simulink model "fixed_graph_sim_lpv"  (R2022b)
settings: Solver=VariableStepAuto  StartTime=0.0  StopTime=80  RelTol=1e-3
values from neighbouring files (symbols this model uses):
  A = [0 1 0; 0 0 1; 0 0 -1/tau]    [cacc_consensus_main.m]    (also in dyn_graph.m; dyn_graph_10.m; dyn_graph_10_disturb.m; fixed_graph.m)
  B = [0 0 1/tau]'    [cacc_consensus_main.m]    (also in dyn_graph.m; dyn_graph_10.m; dyn_graph_10_disturb.m; fixed_graph.m)
  C = diag([1 1 1])    [cacc_consensus_main.m]    (also in dyn_graph.m; dyn_graph_10.m; dyn_graph_10_disturb.m; fixed_graph.m)
  D = [0 0 0]'    [cacc_consensus_main.m]    (also in dyn_graph.m; dyn_graph_10.m; dyn_graph_10_disturb.m; fixed_graph.m)
  h = 1    [cacc_consensus_main.m]    (also in dyn_graph.m; dyn_graph_10.m; dyn_graph_10_disturb.m; fixed_graph.m)
  K_cacc = K_lqr    [cacc_consensus_main.m]    (also in dyn_graph.m = -K_lmi; fixed_graph.m = -K_lmi; fixed_graph_lpv.m = -K_lmi)
  lv = 4.46    [cacc_consensus_main.m]    (also in dyn_graph.m; dyn_graph_10.m; dyn_graph_10_disturb.m; fixed_graph.m)
  q0_init = 0    [cacc_consensus_main.m]    (also in dyn_graph.m; dyn_graph_10.m = rand() * range; dyn_graph_10_disturb.m = rand() * range; fixed_graph.m = rand() * range)
  q1_init = 0    [cacc_consensus_main.m]    (also in dyn_graph.m; dyn_graph_10.m = rand() * range; dyn_graph_10_disturb.m = rand() * range; fixed_graph.m = rand() * range)
  q2_init = 0    [cacc_consensus_main.m]    (also in dyn_graph.m; dyn_graph_10.m = rand() * range; dyn_graph_10_disturb.m = rand() * range; fixed_graph.m = rand() * range)
  q3_init = 0    [cacc_consensus_main.m]    (also in dyn_graph.m; dyn_graph_10.m = rand() * range; dyn_graph_10_disturb.m = rand() * range; fixed_graph.m = rand() * range)
  rv = 0    [cacc_consensus_main.m]    (also in dyn_graph.m; dyn_graph_10.m; dyn_graph_10_disturb.m; fixed_graph.m)
  tau = 0.1    [cacc_consensus_main.m]    (also in dyn_graph.m; dyn_graph_10.m; dyn_graph_10_disturb.m; fixed_graph.m)
libraries: cstblocks x4, simulink x2
settings Model: Creator=phatdo  LastModifiedBy=phatdo
settings DataIOCC: ReturnWorkspaceOutputs=off

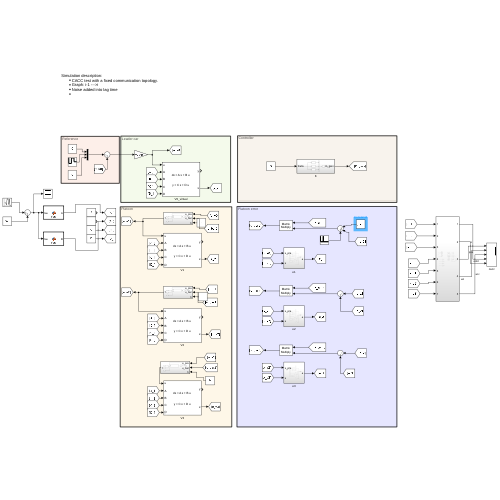
[thumbnail: Simulink's stored preview of the top-level diagram]
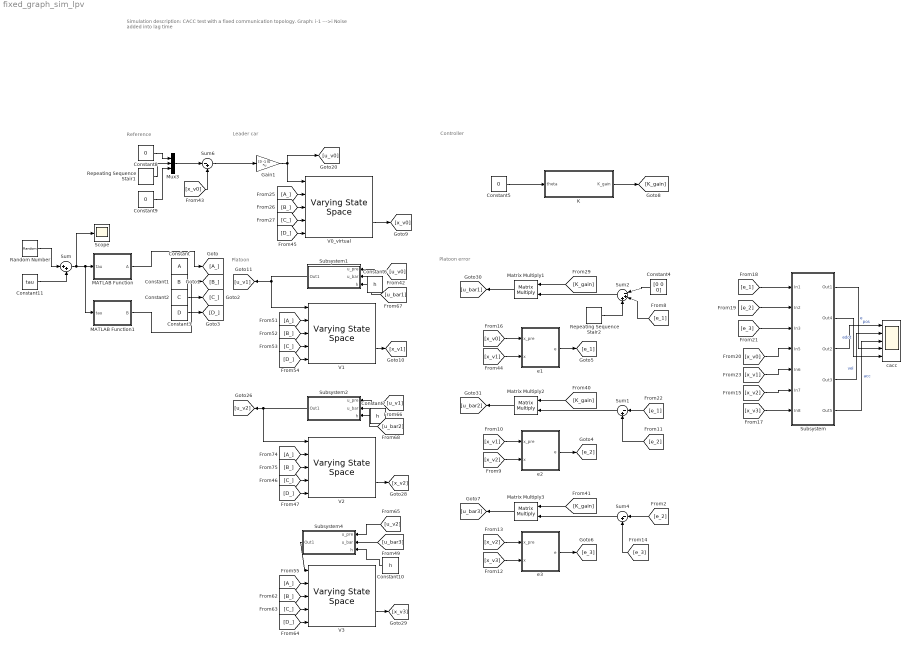
== system fixed_graph_sim_lpv ==
  note: Reference
  note: Controller
  note: Leader car
  note: Platoon
  note: Platoon error
  note: Simulation description:
      | CACC test with a fixed communication topology.
      | Graph: i-1 --->i
      | Noise added into lag time
  Constant : Constant  Value=A
  Constant1 : Constant  Value=B
  Constant10 : Constant  Value=h
  Constant11 : Constant  Value=tau
  Constant2 : Constant  Value=C
  Constant3 : Constant  Value=D
  Constant4 : Constant  Value=[0 0 0]
  Constant5 : Constant  Value=0
  Constant6 : Constant  Value=h
  Constant7 : Constant  Value=h
  Constant8 : Constant  Value=0
  Constant9 : Constant  Value=0
  Gain1 : Gain  Gain=[0 -1 0]  Multiplication=Matrix(K*u) (u vector)
  K : Subsystem
  MATLAB Function : MATLAB Function  TreatAsAtomicUnit=on
  MATLAB Function1 : MATLAB Function  TreatAsAtomicUnit=on
  Matrix Multiply1 : Product  Multiplication=Matrix(*)
  Matrix Multiply2 : Product  Multiplication=Matrix(*)
  Matrix Multiply3 : Product  Multiplication=Matrix(*)
  Mux3 : Mux  Inputs=3
  Random Number : RandomNumber  Variance=0.0001  SampleTime=1
  Repeating Sequence Stair1 : simulink/Sources/Repeating Sequence Stair  OutValues=[5 20 10]  tsamp=20  OutMin=[]  OutMax=[]  OutDataTypeStr=double  OutputDataTypeScalingMode=double  OutDataType=fixdt(0,8)  ConRadixGroup=Best Precision: Vector-wise  OutScaling=2^-12
  Repeating Sequence Stair2 : simulink/Sources/Repeating Sequence Stair  OutValues=[0 0 0 0 0 0 1 0 0 0 0 0 0 0 0 0 0 0].'  tsamp=5  OutMin=[]  OutMax=[]  OutDataTypeStr=double  OutputDataTypeScalingMode=double  OutDataType=fixdt(0,8)  ConRadixGroup=Best Precision: Vector-wise  OutScaling=2^-12
  Scope : Scope
  Subsystem : Subsystem
  Subsystem1 : Subsystem
  Subsystem2 : Subsystem
  Subsystem4 : Subsystem
  Sum : Sum  Inputs=|++
  Sum1 : Sum  Inputs=|-+
  Sum2 : Sum  Inputs=|-++
  Sum4 : Sum  Inputs=|-+
  Sum6 : Sum  Inputs=|-+
  V0_virtual : cstblocks/Linear Parameter Varying/Varying State Space  x0=[q0_init;0;0]  xNames=''  OutputX=on  OutputDX=off
  V1 : cstblocks/Linear Parameter Varying/Varying State Space  x0=[q1_init;0;0]  xNames=''  OutputX=on  OutputDX=off
  V2 : cstblocks/Linear Parameter Varying/Varying State Space  x0=[q2_init;0;0]  xNames=''  OutputX=on  OutputDX=off
  V3 : cstblocks/Linear Parameter Varying/Varying State Space  x0=[q3_init ;0 ; 0]  xNames=''  OutputX=on  OutputDX=off
  cacc : Scope  NumInputPorts=5
  e1 : Subsystem
  e2 : Subsystem
  e3 : Subsystem
  wires:
  Sum2/1 -> Matrix Multiply1/2
  Sum1/1 -> Matrix Multiply2/2
  Constant2/1 -> [C_]
  Constant3/1 -> [D_]
  Constant5/1 -> K/1(theta)
  K/1(K_gain) -> [K_gain]
  [K_gain] -> Matrix Multiply1/1
  [K_gain] -> Matrix Multiply2/1
  [K_gain] -> Matrix Multiply3/1
  Sum4/1 -> Matrix Multiply3/2
  Repeating Sequence Stair1/1 -> Mux3/2
  [A_] -> V1/2
  [C_] -> V1/4
  [D_] -> V0_virtual/5
  V0_virtual/2 -> [x_v0]
  [B_] -> V0_virtual/3
  [A_] -> V0_virtual/2
  V1/2 -> [x_v1]
  Constant9/1 -> Mux3/3
  Constant8/1 -> Mux3/1
  [x_v0] -> Sum6/2
  [C_] -> V0_virtual/4
  [B_] -> V1/3
  Sum6/1 -> Gain1/1
  [D_] -> V3/5
  V3/2 -> [x_v3]
  [A_] -> V3/2
  [B_] -> V3/3
  [u_v1] -> Subsystem2/1(u_pre)
  [C_] -> V2/4
  V2/2 -> [x_v2]
  [D_] -> V2/5
  [C_] -> V3/4
  [A_] -> V2/2
  [B_] -> V2/3
  [x_v0] -> Subsystem/4(In5)
  [x_v1] -> Subsystem/5(In6)
  [x_v2] -> Subsystem/6(In7)
  [x_v3] -> Subsystem/7(In8)
  Subsystem/1(Out1) -> cacc/4  "e"
  Subsystem/3(Out2) -> cacc/1  "pos"
  Subsystem/4(Out3) -> cacc/2  "vel"
  Gain1/1 -> V0_virtual/1, [u_v0]
  Mux3/1 -> Sum6/1
  [u_v0] -> Subsystem1/1(u_pre)
  [u_bar1] -> Subsystem1/2(u_bar)
  [x_v0] -> e1/1(x_pre)
  [x_v1] -> e1/2(x)
  e1/1(e) -> [e_1]
  [e_1] -> Sum2/2
  [x_v1] -> e2/1(x_pre)
  e2/1(e) -> [e_2]
  [x_v2] -> e2/2(x)
  [e_2] -> Sum1/2
  e3/1(e) -> [e_3]
  [x_v3] -> e3/2(x)
  [e_3] -> Sum4/2
  [e_1] -> Subsystem/1(In1)
  [e_2] -> Subsystem/2(In2)
  [e_3] -> Subsystem/3(In3)
  [e_1] -> Sum1/1
  Constant4/1 -> Sum2/1
  Subsystem/2(Out4) -> cacc/5  "edot"
  [D_] -> V1/5
  Subsystem/5(Out5) -> cacc/3  "acc"
  Sum/1 -> Scope/1, MATLAB Function1/1(tau), MATLAB Function/1(tau)
  [u_bar3] -> Subsystem4/2(u_bar)
  [u_v2] -> Subsystem4/1(u_pre)
  [u_bar2] -> Subsystem2/2(u_bar)
  Constant6/1 -> Subsystem1/3(h)
  Constant7/1 -> Subsystem2/3(h)
  Constant10/1 -> Subsystem4/3(h)
  [x_v2] -> e3/1(x_pre)
  Constant11/1 -> Sum/2
  Random Number/1 -> Sum/1
  [e_2] -> Sum4/1
  Matrix Multiply1/1 -> [u_bar1]
  Matrix Multiply2/1 -> [u_bar2]
  Matrix Multiply3/1 -> [u_bar3]
  Subsystem1/1(Out1) -> V1/1, [u_v1]
  Subsystem2/1(Out1) -> V2/1, [u_v2]
  Subsystem4/1(Out1) -> V3/1
  MATLAB Function/1(A) -> [A_]
  MATLAB Function1/1(B) -> [B_]
  Repeating Sequence Stair2/1 -> Sum2/3

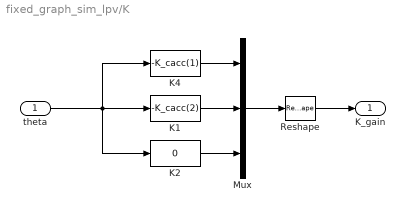
== system fixed_graph_sim_lpv/K ==
  theta : Inport
  K1 : Fcn  Expr=-K_cacc(2)
  K2 : Fcn  Expr=0
  K4 : Fcn  Expr=-K_cacc(1)
  Mux : Mux  Inputs=3
  Reshape : Reshape  OutputDimensionality=Customize  OutputDimensions=[1,3]
  K_gain : Outport
  wires:
  Mux/1 -> Reshape/1
  Reshape/1 -> K_gain/1
  K4/1 -> Mux/1
  K1/1 -> Mux/2
  K2/1 -> Mux/3
  theta/1 -> K2/1, K1/1, K4/1

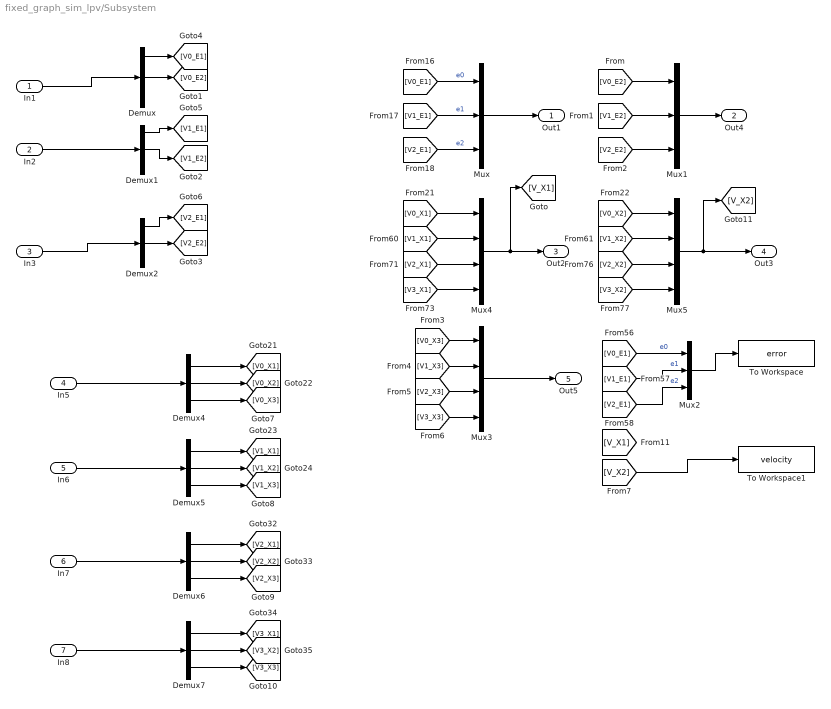
== system fixed_graph_sim_lpv/Subsystem ==
  In1 : Inport
  In2 : Inport  Port=2
  In3 : Inport  Port=3
  In5 : Inport  Port=4
  In6 : Inport  Port=5
  In7 : Inport  Port=6
  In8 : Inport  Port=7
  Demux{,1..2,4..7} (7 alike) : Demux  Outputs=3
  Mux : Mux  Inputs=3
  Mux1 : Mux  Inputs=3
  Mux2 : Mux  Inputs=3
  Mux3 : Mux
  Mux4 : Mux
  Mux5 : Mux
  To Workspace : ToWorkspace  VariableName=error  SaveFormat=Timeseries  SampleTime=-1
  To Workspace1 : ToWorkspace  VariableName=velocity  SaveFormat=Timeseries  SampleTime=-1
  Out1 : Outport
  Out4 : Outport  Port=2
  Out2 : Outport  Port=3
  Out3 : Outport  Port=4
  Out5 : Outport  Port=5
  wires:
  [V2_X1] -> Mux4/3
  Demux/1 -> [V0_E1]
  Demux2/1 -> [V2_E1]
  In2/1 -> Demux1/1
  [V2_E1] -> Mux2/3  "e2"
  [V0_X1] -> Mux4/1
  Demux1/1 -> [V1_E1]
  [V3_X1] -> Mux4/4
  Demux6/2 -> [V2_X2]
  Demux7/1 -> [V3_X1]
  Demux4/1 -> [V0_X1]
  Demux4/2 -> [V0_X2]
  In7/1 -> Demux6/1
  Demux5/2 -> [V1_X2]
  Demux6/1 -> [V2_X1]
  In8/1 -> Demux7/1
  [V1_X2] -> Mux5/2
  In1/1 -> Demux/1
  [V1_E1] -> Mux2/2  "e1"
  [V0_E1] -> Mux2/1  "e0"
  Mux4/1 -> [V_X1], Out2/1
  [V3_X2] -> Mux5/4
  [V2_X2] -> Mux5/3
  [V0_X2] -> Mux5/1
  Demux7/2 -> [V3_X2]
  [V1_E1] -> Mux/2  "e1"
  In5/1 -> Demux4/1
  [V1_X1] -> Mux4/2
  In6/1 -> Demux5/1
  [V2_E1] -> Mux/3  "e2"
  [V0_E1] -> Mux/1  "e0"
  Mux/1 -> Out1/1
  In3/1 -> Demux2/1
  Demux5/1 -> [V1_X1]
  Demux/2 -> [V0_E2]
  Demux1/2 -> [V1_E2]
  Demux2/2 -> [V2_E2]
  [V0_E2] -> Mux1/1
  [V1_E2] -> Mux1/2
  [V2_E2] -> Mux1/3
  Mux1/1 -> Out4/1
  Demux4/3 -> [V0_X3]
  Demux5/3 -> [V1_X3]
  Demux6/3 -> [V2_X3]
  Demux7/3 -> [V3_X3]
  [V0_X3] -> Mux3/1
  [V1_X3] -> Mux3/2
  [V2_X3] -> Mux3/3
  [V3_X3] -> Mux3/4
  Mux3/1 -> Out5/1
  [V_X2] -> To Workspace1/1
  Mux5/1 -> [V_X2], Out3/1
  Mux2/1 -> To Workspace/1

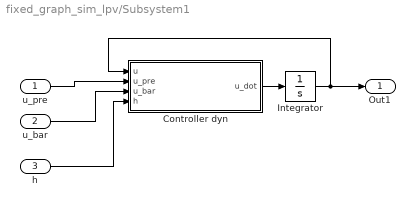
== system fixed_graph_sim_lpv/Subsystem1 ==
  u_pre : Inport
  u_bar : Inport  Port=2
  h : Inport  Port=3
  Controller dyn : MATLAB Function  TreatAsAtomicUnit=on
  Integrator : Integrator
  Out1 : Outport
  wires:
  Controller dyn/1(u_dot) -> Integrator/1
  Integrator/1 -> Controller dyn/1(u), Out1/1
  u_pre/1 -> Controller dyn/2(u_pre)
  u_bar/1 -> Controller dyn/3(u_bar)
  h/1 -> Controller dyn/4(h)

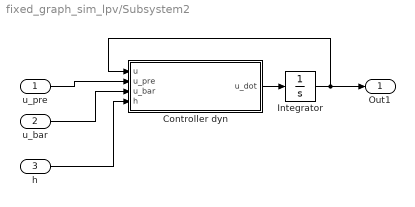
== system fixed_graph_sim_lpv/Subsystem2 ==
  u_pre : Inport
  u_bar : Inport  Port=2
  h : Inport  Port=3
  Controller dyn : MATLAB Function  TreatAsAtomicUnit=on
  Integrator : Integrator
  Out1 : Outport
  wires:
  Controller dyn/1(u_dot) -> Integrator/1
  Integrator/1 -> Controller dyn/1(u), Out1/1
  u_pre/1 -> Controller dyn/2(u_pre)
  u_bar/1 -> Controller dyn/3(u_bar)
  h/1 -> Controller dyn/4(h)

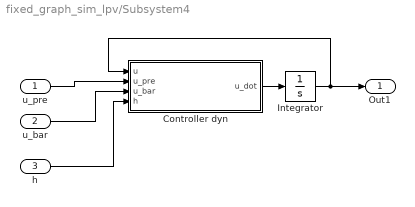
== system fixed_graph_sim_lpv/Subsystem4 ==
  u_pre : Inport
  u_bar : Inport  Port=2
  h : Inport  Port=3
  Controller dyn : MATLAB Function  TreatAsAtomicUnit=on
  Integrator : Integrator
  Out1 : Outport
  wires:
  Controller dyn/1(u_dot) -> Integrator/1
  Integrator/1 -> Controller dyn/1(u), Out1/1
  u_pre/1 -> Controller dyn/2(u_pre)
  u_bar/1 -> Controller dyn/3(u_bar)
  h/1 -> Controller dyn/4(h)

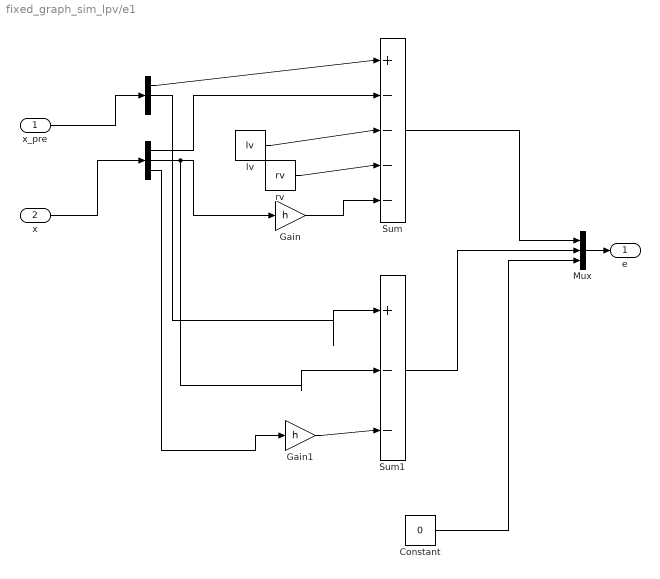
== system fixed_graph_sim_lpv/e1 ==
  x_pre : Inport
  x : Inport  Port=2
  " " : Demux  Outputs=3
  "   " : Demux  Outputs=3
  Constant : Constant  Value=0
  Gain : Gain  Gain=h
  Gain1 : Gain  Gain=h
  Mux : Mux  Inputs=3
  Sum : Sum  Inputs=|+----
  Sum1 : Sum  Inputs=|+--
  lv : Constant  Value=lv
  rv : Constant  Value=rv
  e : Outport
  wires:
  " "/1 -> Sum/1
  "   "/1 -> Sum/2
  lv/1 -> Sum/3
  rv/1 -> Sum/4
  Gain/1 -> Sum/5
  Sum/1 -> Mux/1
  "   "/2 -> Sum1/2, Gain/1
  " "/2 -> Sum1/1
  "   "/3 -> Gain1/1
  Gain1/1 -> Sum1/3
  x_pre/1 -> " "/1
  x/1 -> "   "/1
  Constant/1 -> Mux/3
  Mux/1 -> e/1
  Sum1/1 -> Mux/2

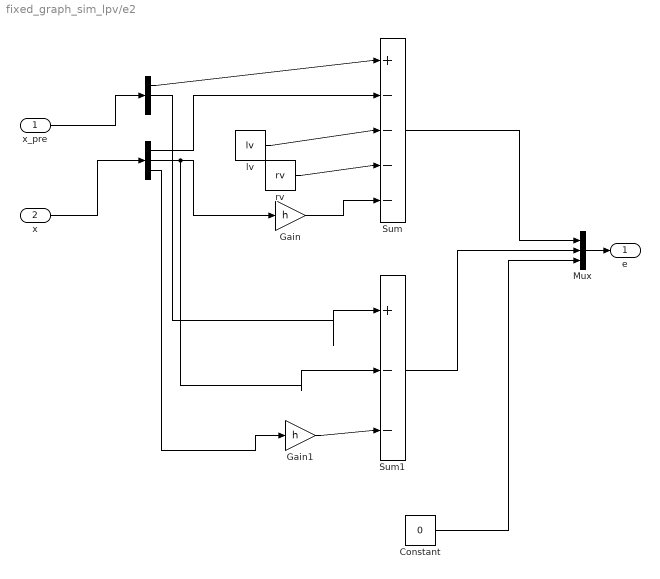
== system fixed_graph_sim_lpv/e2 ==
  x_pre : Inport
  x : Inport  Port=2
  " " : Demux  Outputs=3
  "   " : Demux  Outputs=3
  Constant : Constant  Value=0
  Gain : Gain  Gain=h
  Gain1 : Gain  Gain=h
  Mux : Mux  Inputs=3
  Sum : Sum  Inputs=|+----
  Sum1 : Sum  Inputs=|+--
  lv : Constant  Value=lv
  rv : Constant  Value=rv
  e : Outport
  wires:
  " "/1 -> Sum/1
  "   "/1 -> Sum/2
  lv/1 -> Sum/3
  rv/1 -> Sum/4
  Gain/1 -> Sum/5
  Sum/1 -> Mux/1
  "   "/2 -> Sum1/2, Gain/1
  " "/2 -> Sum1/1
  "   "/3 -> Gain1/1
  Gain1/1 -> Sum1/3
  x_pre/1 -> " "/1
  x/1 -> "   "/1
  Constant/1 -> Mux/3
  Mux/1 -> e/1
  Sum1/1 -> Mux/2

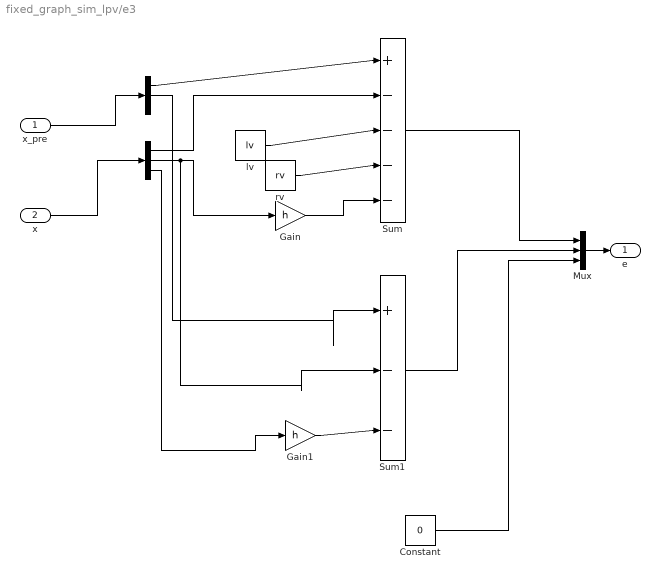
== system fixed_graph_sim_lpv/e3 ==
  x_pre : Inport
  x : Inport  Port=2
  " " : Demux  Outputs=3
  "   " : Demux  Outputs=3
  Constant : Constant  Value=0
  Gain : Gain  Gain=h
  Gain1 : Gain  Gain=h
  Mux : Mux  Inputs=3
  Sum : Sum  Inputs=|+----
  Sum1 : Sum  Inputs=|+--
  lv : Constant  Value=lv
  rv : Constant  Value=rv
  e : Outport
  wires:
  Sum1/1 -> Mux/2
  Mux/1 -> e/1
  Constant/1 -> Mux/3
  x/1 -> "   "/1
  x_pre/1 -> " "/1
  Gain1/1 -> Sum1/3
  "   "/3 -> Gain1/1
  " "/2 -> Sum1/1
  "   "/2 -> Gain/1, Sum1/2
  Sum/1 -> Mux/1
  Gain/1 -> Sum/5
  rv/1 -> Sum/4
  lv/1 -> Sum/3
  "   "/1 -> Sum/2
  " "/1 -> Sum/1

== matlab function fixed_graph_sim_lpv/Subsystem1/Controller dyn ==
  data: u input; u_dot output; u_pre input; u_bar input; h input
function u_dot = cacc(u, u_pre, u_bar,h)

h = h; % second

u_dot = -1/h * u + 1/h * (u_pre - u_bar);

end

== matlab function fixed_graph_sim_lpv/MATLAB Function ==
  data: tau input; A output
function A = fcn(tau)

A = [0 1 0; 0 0 1; 0 0 -1/tau];

end

== matlab function fixed_graph_sim_lpv/Subsystem2/Controller dyn ==
  data: u input; u_dot output; u_pre input; u_bar input; h input
function u_dot = cacc(u, u_pre, u_bar,h)

h = h; % second

u_dot = -1/h * u + 1/h * (u_pre - u_bar);

end

== matlab function fixed_graph_sim_lpv/MATLAB Function1 ==
  data: tau input; B output
function B = fcn(tau)

B = [0; 0; 1/tau];

end

== matlab function fixed_graph_sim_lpv/Subsystem4/Controller dyn ==
  data: u input; u_dot output; u_pre input; u_bar input; h input
function u_dot = cacc(u, u_pre, u_bar,h)

h = h; % second

u_dot = -1/h * u + 1/h * (u_pre - u_bar);

end
